simulink model "test_model_sw_only"  (R2018a)
settings: Solver=VariableStepAuto  StartTime=0.0  StopTime=10.0  RelTol=1e-3
settings Model: Creator=streit  LastModifiedBy=puya
settings CodeAppCC: StateflowObjectComments=on

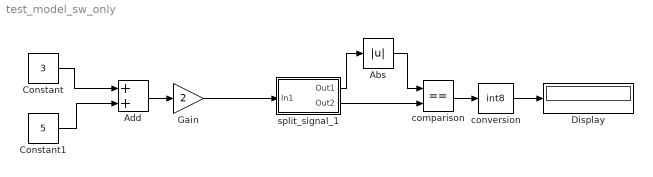
== system test_model_sw_only ==
  Abs : Abs  Tag=sw
  Add : Sum  Tag=sw
  Constant : Constant  Value=3
  Constant1 : Constant  Value=5
  Display : Display
  Gain : Gain  Tag=sw  Gain=2
  comparison : RelationalOperator  Tag=sw  Operator===  OutDataTypeStr=boolean  RndMeth=Simplest
  conversion : DataTypeConversion  Tag=sw  OutDataTypeStr=int8
  split_signal_1 : Subsystem  Tag=sw
  wires:
  Constant/1 -> Add/1
  comparison/1 -> conversion/1
  split_signal_1/2(Out2) -> comparison/2
  split_signal_1/1(Out1) -> Abs/1
  conversion/1 -> Display/1
  Gain/1 -> split_signal_1/1(In1)
  Constant1/1 -> Add/2
  Abs/1 -> comparison/1
  Add/1 -> Gain/1

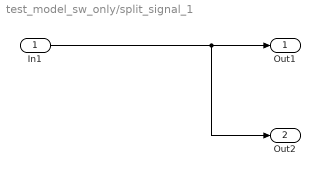
== system test_model_sw_only/split_signal_1 ==
  In1 : Inport
  Out1 : Outport
  Out2 : Outport  Port=2
  wires:
  In1/1 -> Out2/1, Out1/1
